simulink model "video"  (Simulink 7.7)
settings: Solver=ode45  StartTime=0.0  StopTime=10.0  RelTol=1e-3
undefined symbols (not defined in the file or in its folder): jet
libraries: vipsnks x1, dspsrcs4 x1
settings Model: Creator=katsikas  LastModifiedBy=katsikas

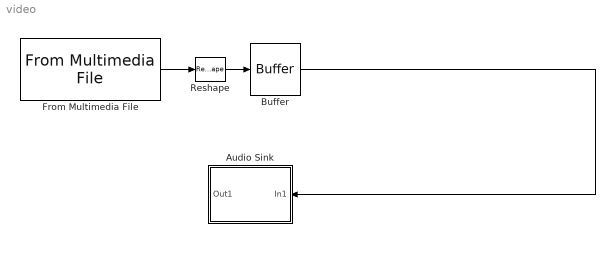
== system video ==
  Audio Sink : Subsystem
  Buffer : Buffer  N=188  TreatMby1Signals=One channel
  From Multimedia File : dspsrcs4/From Multimedia File  inputFilename=/usr/local/MATLAB/R2011a/toolbox/vision/visiondemos/vipmen.avi  loop=on  numPlays=inf  outputStreams=Video only  videoDataType=uint8  audioDataType=int16  inheritSampleTime=on  userDefinedSampleTime=1/30  noAudioOutput=off  isIntensityVideo=off  fourcc=Intensity  colorVideoFormat=Separate color signals  outputEOF=off  dataOrg=Column-major  audioFrameSize=1024  computeAudioFrameSize=off
  Reshape : Reshape
  wires:
  From Multimedia File/1 -> Reshape/1
  Reshape/1 -> Buffer/1
  Buffer/1 -> Audio Sink/1(In1)

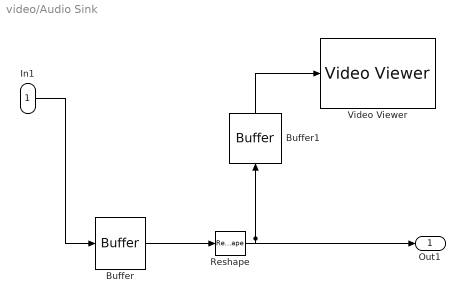
== system video/Audio Sink ==
  In1 : Inport
  Buffer : Buffer  N=120*160  TreatMby1Signals=One channel
  Buffer1 : Buffer  N=120  TreatMby1Signals=One channel
  Reshape : Reshape  OutputDimensionality=Customize  OutputDimensions=[120,160]
  Video Viewer : vipsnks/Video Viewer  inputType=Obsolete7b  imagePorts=One multidimensional signal  useColorMap=off  colormapValue=jet(256)  specRange=off  minInputVal=0  maxInputVal=255  FigPos=[379 549 320 188]  AxisZoom=on  trueSizedOnce=off  OpenAtMdlStart=on
  Out1 : Outport
  wires:
  In1/1 -> Buffer/1
  Buffer/1 -> Reshape/1
  Reshape/1 -> Out1/1, Buffer1/1
  Buffer1/1 -> Video Viewer/1
